simulink model "sfcndemo_dsfunc"  (Simulink 6.0)
settings: Solver=FixedStepDiscrete  StartTime=0.0  StopTime=10.0  RelTol=1e-3
settings Model: Creator=The MathWorks Inc.  LastModifiedBy=batserve  ExtModeTrigMode=oneshot  ExtModeArmWhenConnect=off  ExtModeAutoUpdateStatusClock=off
settings DataIOCC: LimitDataPoints=off
settings OptimizationCC: BooleanDataType=off
settings DebuggingCC: CheckExecutionContextPreStartOutputMsg=on  CheckExecutionContextRuntimeOutputMsg=on  SolverPrmCheckMsg=none
settings HardwareCC: TargetUnknown=on

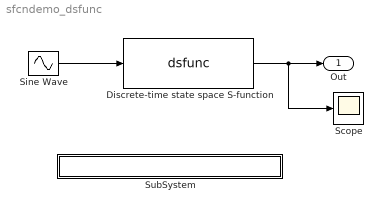
== system sfcndemo_dsfunc ==
  "Discrete-time state space S-function " : S-Function  FunctionName=dsfunc
      mask Type: S-function: dsfunc
      mask Description: This is a S-function which does the discrete state space system.
      mask Display: disp('x(n+1) = Ax(n) + Bu(n)\n y(n)     = Cx(n) + Du(n) ');
  Scope : Scope
      settings: TimeRange=10  YMin=-80  YMax=60
  Sine Wave : Sin  Amplitude=[1 2]  SampleTime=0
  SubSystem : Subsystem  PropExecContextAcrossSSBoundary=on
      settings: OpenFcn=edit(fullfile(matlabroot,'simulink','src','dsfunc.c'))
      mask Display: disp('matlabroot\simulink\src\dsfunc.c');
  Out : Outport  InitialOutput=0
  wires:
  Sine Wave/1 -> "Discrete-time state space S-function "/1
  "Discrete-time state space S-function "/1 -> Out/1, Scope/1

== system sfcndemo_dsfunc/SubSystem ==
